simulink model "MSFartoystyring_PathFollowing"  (R2019a)
settings: Solver=ode45  StartTime=tstart  StopTime=tstop  RelTol=1e-3  EnableMultiTasking=on
values from neighbouring files (symbols this model uses):
  a1 = 6145    [run.m]
  a2 = -0.0075    [run.m]
  a3 = 1.0384    [run.m]
  c = 1    [run.m]
  delta = 0.8    [run.m]
  K_d = (2*zeta*omega_n*T-1) / K    [Task_Parameters.m]    (also in run.m = -161.6429)
  K_i = (omega_n^3*T) /(10*K)    [Task_Parameters.m]    (also in run.m = -0.0023)
  K_p = omega_n^2*T / K    [Task_Parameters.m]    (also in run.m = -2.2816)
  K_u_i = 1e-5    (= 1e-05)    [run.m]
  K_u_p = 0.2    [run.m]
  omega = 0.05    [run.m]
  p0 = zeros(1000,700)    [run.m]
  psi0 = 60*d2r    (= 1.0471975512)    [run.m]
  r0 = 0    [run.m]
  tsamp = 10    [run.m]
  v0 = [6.63 0]'    [run.m]
undefined symbols (not defined in the file or in its folder): msfartoystyring
settings Model: ExtModeAutoUpdateStatusClock=off  Creator=christh  LastModifiedBy=zhy
settings DataIOCC: LimitDataPoints=on  SaveFormat=Array  ReturnWorkspaceOutputs=off
settings OptimizationCC: ExpressionDepthLimit=2147483647  InitFltsAndDblsToZero=on  LifeSpan=inf
settings DebuggingCC: UnderspecifiedInitializationDetection=Classic  MergeDetectMultiDrivingBlocksExec=none  SolverPrmCheckMsg=warning  FcnCallInpInsideContextMsg=warning  StateNameClashWarn=warning  PregeneratedLibrarySubsystemCodeDiagnostic=none  SFUnexpectedBacktrackingDiag=warning  SFNoUnconditionalDefaultTransitionDiag=warning  SFExecutionAtInitializationDiag=none  ArithmeticOperatorsInVariantConditions=warning
settings HardwareCC: ProdBitPerPointer=32  ProdBitPerSizeT=32  ProdBitPerPtrDiffT=32  ProdLargestAtomicFloat=None  ProdIntDivRoundTo=Undefined  ProdEndianess=Unspecified  ProdWordSize=32  ProdHWDeviceType=32-bit Generic
settings ModelReferenceCC: PropagateSignalLabelsOutOfModel=off
settings SFSimCC: SimUseLocalCustomCode=off
settings RTWCC: RTWUseLocalCustomCode=off
settings CodeAppCC: StateflowObjectComments=on
settings GRTTargetCC: TargetLangStandard=C89/C90 (ANSI)  GeneratePreprocessorConditionals=Disable all  CombineOutputUpdateFcns=off  GRTInterface=on
settings ConfigComp: CovMetricSettings=dw  CovHtmlReporting=on  CovSaveCumulativeToWorkspaceVar=on  CovSaveSingleToWorkspaceVar=on  CovExternalEMLEnable=off

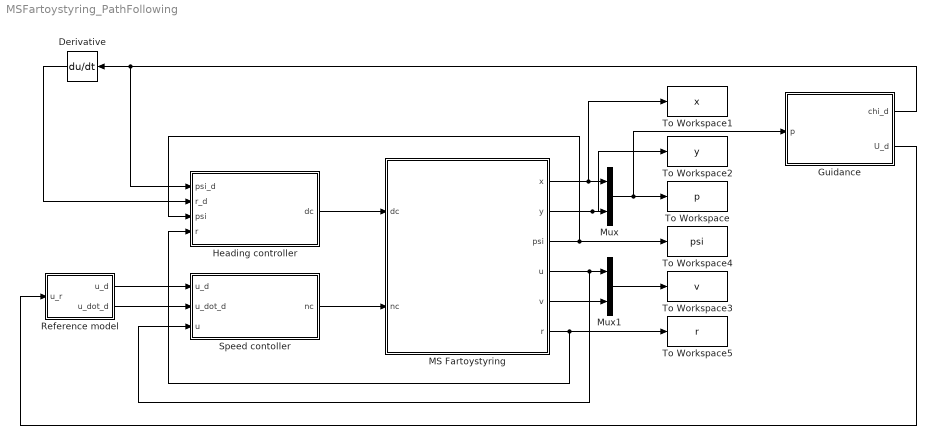
== system MSFartoystyring_PathFollowing ==
  Derivative : Derivative
  Guidance : MATLAB Function  TreatAsAtomicUnit=on
  Heading controller : Subsystem
  MS Fartoystyring : Subsystem  mask(MS Fartoystyring for Assignment 3 G&C){x0=p0(1), y0=p0(2), u0=v0(1), v0=v0(2), psi0=psi0, r0=r0, c=c}
      mask prompts: x0 "x(t0) (m)"; y0 "y(t0) (m)"; u0 "u(t0) (m/s)"; v0 "v(t0) (m/s)"; psi0 "psi(t0) (rad)"; r0 "r(t0) (rad/s)"; c "current (0 or 1)"
      mask help:
      | Block corresponding to Figure 1 in the assignment text. Gives the response of the ship.
      |
      | The design speed of MS Fartoystyring is u=8.23 m/s.
      |
      | Input:
      | dc: commanded rudder (rad), dmax=25*pi/180
      | nc: commanded shaft speed (rad/s), nmax=85*2*pi/60
      |
      | Output:
      | x: north pos (m)
      | y: east pos (m)
      | u: surge (m/s)
      | v: sway (m/s)
      | psi: heading (rad)
      | r: yaw (rad/s)
      mask Help: Comments, bugs and help requests can be directed to the TA. Email on course website.
  Mux : Mux  Inputs=2
  Mux1 : Mux  Inputs=2
  Reference model : Subsystem
  Speed contoller : Subsystem
  To Workspace : ToWorkspace  VariableName=p  SaveFormat=Timeseries  SampleTime=tsamp
  To Workspace1 : ToWorkspace  VariableName=x  SampleTime=tsamp
  To Workspace2 : ToWorkspace  VariableName=y  SampleTime=tsamp
  To Workspace3 : ToWorkspace  VariableName=v  SaveFormat=Timeseries  SampleTime=tsamp
  To Workspace4 : ToWorkspace  VariableName=psi  SampleTime=tsamp
  To Workspace5 : ToWorkspace  VariableName=r  SaveFormat=Timeseries  SampleTime=tsamp
  wires:
  MS Fartoystyring/1(x) -> To Workspace1/1, Mux/1
  MS Fartoystyring/2(y) -> To Workspace2/1, Mux/2
  MS Fartoystyring/4(u) -> Speed contoller/3(u), Mux1/1
  MS Fartoystyring/5(v) -> Mux1/2
  Mux/1 -> Guidance/1(p), To Workspace/1
  Mux1/1 -> To Workspace3/1
  MS Fartoystyring/3(psi) -> Heading controller/3(psi), To Workspace4/1
  MS Fartoystyring/6(r) -> Heading controller/4(r), To Workspace5/1
  Speed contoller/1(nc) -> MS Fartoystyring/2(nc)
  Heading controller/1(dc) -> MS Fartoystyring/1(dc)
  Reference model/1(u_d) -> Speed contoller/1(u_d)
  Reference model/2(u_dot_d) -> Speed contoller/2(u_dot_d)
  Guidance/1(chi_d) -> Heading controller/1(psi_d), Derivative/1
  Derivative/1 -> Heading controller/2(r_d)
  Guidance/2(U_d) -> Reference model/1(u_r)

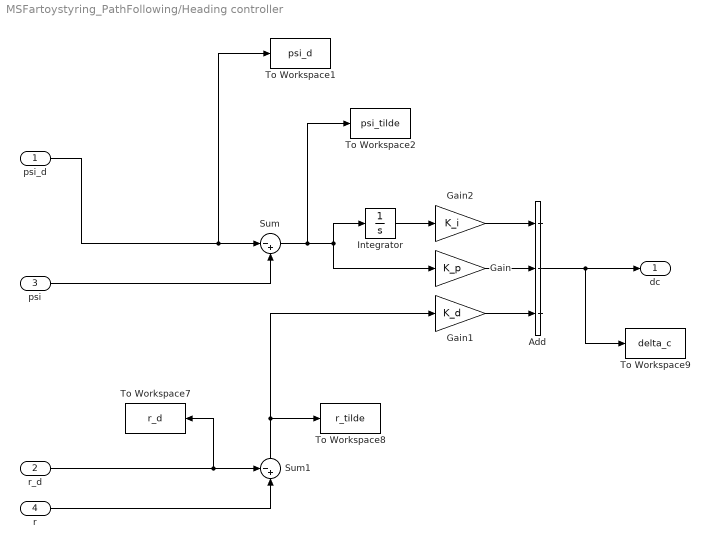
== system MSFartoystyring_PathFollowing/Heading controller ==
  psi_d : Inport
  r_d : Inport  Port=2
  psi : Inport  Port=3
  r : Inport  Port=4
  Add : Sum  Inputs=---
  Gain : Gain  Gain=K_p
  Gain1 : Gain  Gain=K_d
  Gain2 : Gain  Gain=K_i
  Integrator : Integrator
  Sum : Sum  Inputs=|-+
  Sum1 : Sum  Inputs=-+|
  To Workspace1 : ToWorkspace  VariableName=psi_d  SaveFormat=Timeseries  SampleTime=-1
  To Workspace2 : ToWorkspace  VariableName=psi_tilde  SaveFormat=Timeseries  SampleTime=-1
  To Workspace7 : ToWorkspace  VariableName=r_d  SaveFormat=Timeseries  SampleTime=-1
  To Workspace8 : ToWorkspace  VariableName=r_tilde  SaveFormat=Timeseries  SampleTime=-1
  To Workspace9 : ToWorkspace  VariableName=delta_c  SaveFormat=Timeseries  SampleTime=-1
  dc : Outport
  wires:
  Sum1/1 -> Gain1/1, To Workspace8/1
  Gain2/1 -> Add/1
  Gain/1 -> Add/2
  r_d/1 -> To Workspace7/1, Sum1/1
  psi/1 -> Sum/2
  Integrator/1 -> Gain2/1
  Sum/1 -> To Workspace2/1, Integrator/1, Gain/1
  Gain1/1 -> Add/3
  psi_d/1 -> To Workspace1/1, Sum/1
  Add/1 -> To Workspace9/1, dc/1
  r/1 -> Sum1/2

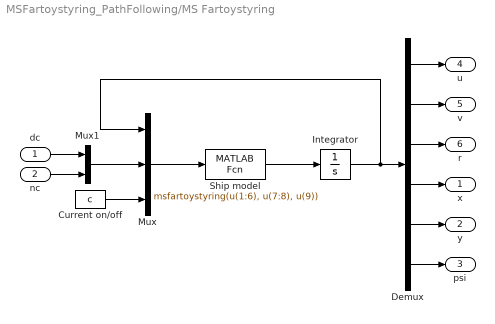
== system MSFartoystyring_PathFollowing/MS Fartoystyring ==
  dc : Inport
  nc : Inport  Port=2
  Current on/off : Constant  Value=c
  Demux : Demux  Outputs=6
  Integrator : Integrator  InitialCondition=[u0 v0 r0 x0 y0 psi0]'
  Mux : Mux  Inputs=3
  Mux1 : Mux  Inputs=2
  Ship model : MATLABFcn  MATLABFcn=msfartoystyring(u(1:6), u(7:8), u(9))  OutputDimensions=6
  x : Outport
  y : Outport  Port=2
  psi : Outport  Port=3
  u : Outport  Port=4
  v : Outport  Port=5
  r : Outport  Port=6
  wires:
  Integrator/1 -> Mux/1, Demux/1
  Mux1/1 -> Mux/2
  dc/1 -> Mux1/1
  nc/1 -> Mux1/2
  Demux/1 -> u/1
  Demux/2 -> v/1
  Demux/3 -> r/1
  Demux/4 -> x/1
  Demux/5 -> y/1
  Demux/6 -> psi/1
  Current on/off/1 -> Mux/3
  Ship model/1 -> Integrator/1
  Mux/1 -> Ship model/1

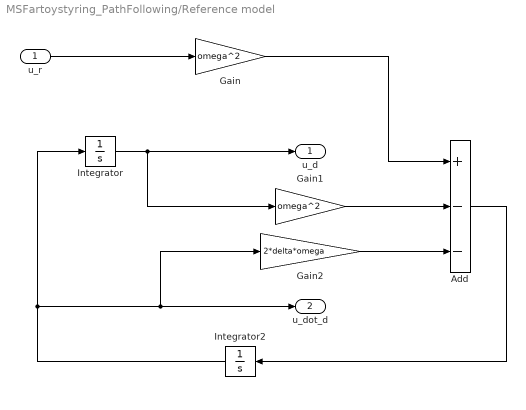
== system MSFartoystyring_PathFollowing/Reference model ==
  u_r : Inport
  Add : Sum  Inputs=+--
  Gain : Gain  Gain=omega^2
  Gain1 : Gain  Gain=omega^2
  Gain2 : Gain  Gain=2*delta*omega
  Integrator : Integrator
  Integrator2 : Integrator
  u_d : Outport
  u_dot_d : Outport  Port=2
  wires:
  u_r/1 -> Gain/1
  Integrator/1 -> u_d/1, Gain1/1
  Integrator2/1 -> Gain2/1, u_dot_d/1, Integrator/1
  Gain1/1 -> Add/2
  Gain2/1 -> Add/3
  Gain/1 -> Add/1
  Add/1 -> Integrator2/1

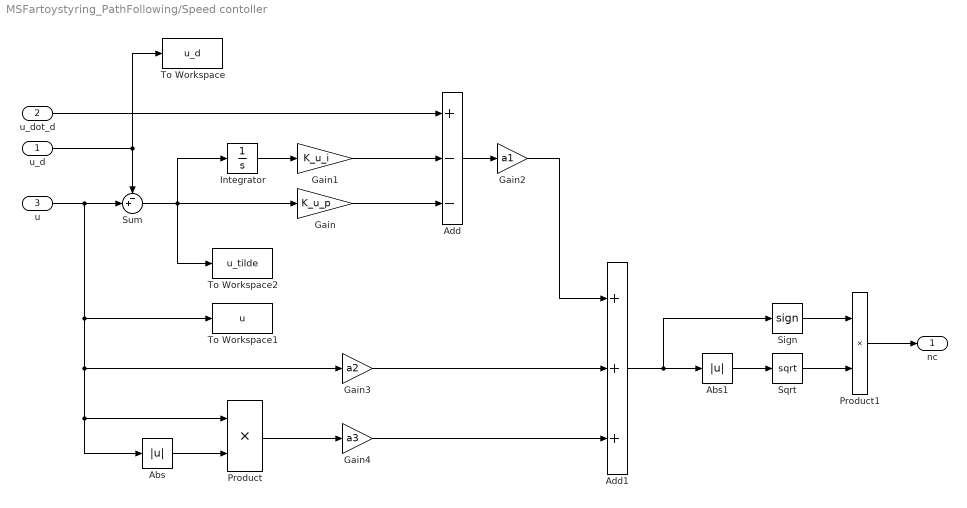
== system MSFartoystyring_PathFollowing/Speed contoller ==
  u_d : Inport
  u_dot_d : Inport  Port=2
  u : Inport  Port=3
  Abs : Abs
  Abs1 : Abs
  Add : Sum  Inputs=+--
  Add1 : Sum  Inputs=+++
  Gain : Gain  Gain=K_u_p
  Gain1 : Gain  Gain=K_u_i
  Gain2 : Gain  Gain=a1
  Gain3 : Gain  Gain=a2
  Gain4 : Gain  Gain=a3
  Integrator : Integrator
  Product : Product
  Product1 : Product
  Sign : Signum
  Sqrt : Sqrt  SaturateOnIntegerOverflow=on
  Sum : Sum  Inputs=-+|
  To Workspace : ToWorkspace  VariableName=u_d  SaveFormat=Timeseries  SampleTime=-1
  To Workspace1 : ToWorkspace  VariableName=u  SaveFormat=Timeseries  SampleTime=-1
  To Workspace2 : ToWorkspace  VariableName=u_tilde  SaveFormat=Timeseries  SampleTime=-1
  nc : Outport
  wires:
  u/1 -> Product/1, Abs/1, Gain3/1, To Workspace1/1, Sum/2
  u_d/1 -> Sum/1, To Workspace/1
  Sum/1 -> Integrator/1, To Workspace2/1, Gain/1
  Integrator/1 -> Gain1/1
  Add/1 -> Gain2/1
  Abs/1 -> Product/2
  Product/1 -> Gain4/1
  Gain3/1 -> Add1/2
  Gain4/1 -> Add1/3
  Gain2/1 -> Add1/1
  Add1/1 -> Sign/1, Abs1/1
  Abs1/1 -> Sqrt/1
  Sqrt/1 -> Product1/2
  Sign/1 -> Product1/1
  Product1/1 -> nc/1
  Gain1/1 -> Add/2
  Gain/1 -> Add/3
  u_dot_d/1 -> Add/1

== matlab function MSFartoystyring_PathFollowing/Guidance ==
  settings: updateMethod=DISCRETE
  data: chi_d output; U_d output; p input
function [chi_d,U_d]= fcn(p)

persistent k;
persistent WP;
persistent x_k;
persistent y_k;
persistent x_k_1;
persistent y_k_1;

x_t = p(1);
y_t = p(2);

if isempty(k)
   WP = [0,-3500,-7000,-12000,-15000,-18000;0,-2500,-500,-3500,-500,-2000];
   k = 1;
   x_k = WP(1,k);
   y_k = WP(2,k);
   x_k_1 = WP(1,k+1);
   y_k_1 = WP(2,k+1);
end
 
R_distantce = sqrt((x_t-x_k_1)^2+(y_t-y_k_1)^2);

if k<5
    if R_distantce<500
        k = k+1; 
        x_k = WP(1,k);
        y_k = WP(2,k);
        x_k_1 = WP(1,k+1);
        y_k_1 = WP(2,k+1);
    end 
else
        x_k = WP(1,5);
        y_k = WP(2,5);
        x_k_1 = WP(1,6);
        y_k_1 = WP(2,6);
end

if x_k_1-x_k<0
    alpha_k = atan((y_k_1-y_k)/(x_k_1-x_k))+pi;
else
    alpha_k = atan((y_k_1-y_k)/(x_k_1-x_k))
end

e = -(x_t-x_k)*sin(alpha_k) + (y_t-y_k)*cos(alpha_k);
delta = 500;
chi_r = atan(-e/delta);
chi_k = alpha_k;
chi_d = chi_r + chi_k;

U_d = 5;
